simulink model "inloop_tf_model_spring"  (R2020b)
settings: Solver=VariableStepAuto  StartTime=0.0  StopTime=10.0  RelTol=1e-3
undefined symbols (not defined in the file or in its folder): b, ct, g, Jm, Ke, Kt, L, m, Rm
libraries: shared6dof x1
settings Model: Creator=Josh_  LastModifiedBy=Josh_

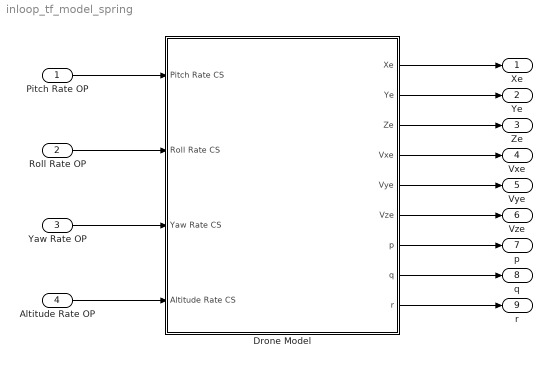
== system inloop_tf_model_spring ==
  Pitch Rate OP : Inport
  Roll Rate OP : Inport  Port=2
  Yaw Rate OP : Inport  Port=3
  Altitude Rate OP : Inport  Port=4
  Drone Model : Subsystem
  Xe : Outport
  Ye : Outport  Port=2
  Ze : Outport  Port=3
  Vxe : Outport  Port=4
  Vye : Outport  Port=5
  Vze : Outport  Port=6
  p : Outport  Port=7
  q : Outport  Port=8
  r : Outport  Port=9
  wires:
  Pitch Rate OP/1 -> Drone Model/1(Pitch Rate CS)
  Drone Model/9(r) -> r/1
  Roll Rate OP/1 -> Drone Model/2(Roll Rate CS)
  Drone Model/7(p) -> p/1
  Drone Model/4(Vxe) -> Vxe/1
  Drone Model/2(Ye) -> Ye/1
  Drone Model/3(Ze) -> Ze/1
  Altitude Rate OP/1 -> Drone Model/4(Altitude Rate CS)
  Drone Model/8(q) -> q/1
  Drone Model/6(Vze) -> Vze/1
  Drone Model/5(Vye) -> Vye/1
  Drone Model/1(Xe) -> Xe/1
  Yaw Rate OP/1 -> Drone Model/3(Yaw Rate CS)

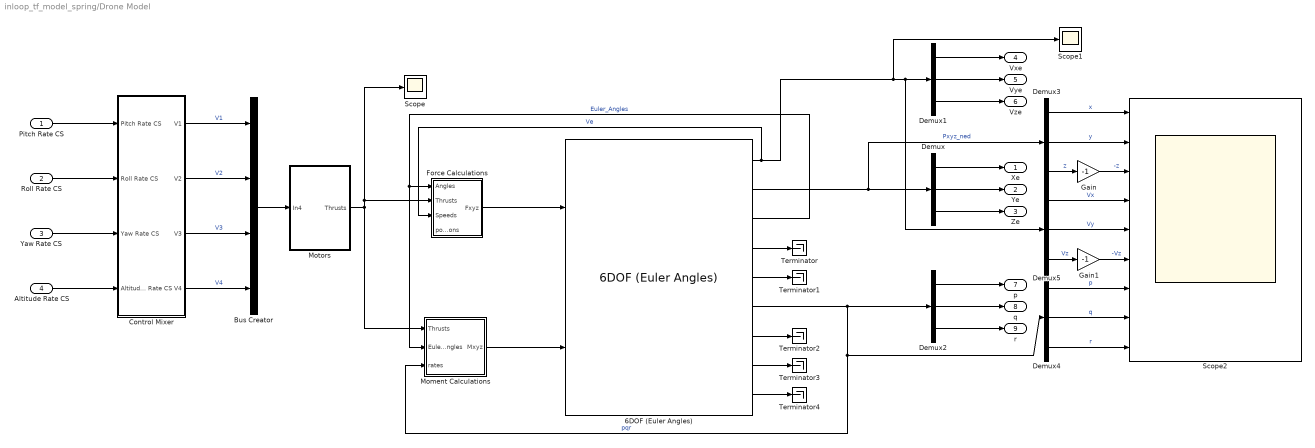
== system inloop_tf_model_spring/Drone Model ==
  Pitch Rate CS : Inport
  Roll Rate CS : Inport  Port=2
  Yaw Rate CS : Inport  Port=3
  Altitude Rate CS : Inport  Port=4
  6DOF (Euler Angles) : shared6dof/6DOF (Euler Angles)  units=Metric (MKS)  mtype=Fixed  rep=Euler Angles  xme_0=[0 0 0]  Vm_0=[0 0 0]  eul_0=[0 0 0]  pm_0=[0 0 0]  mass_0=m  mass_e=0.5  mass_f=2.0  inertia=eye(3)  inertia_e=eye(3)  inertia_f=2*eye(3)  k_quat=1.0  vre_flag=on  abi_flag=on  aMode=0  xme_statename=''  Vm_statename=''  eul_statename=''  quat_statename=''  pm_statename=''  mass_statename=''
      settings: SourceProductBaseCode=AE,PW,MT,UV,VE,VP
  Bus Creator : BusCreator  Inputs=4
  Control Mixer : Subsystem
  Demux{,1..5} (6 alike) : Demux  Outputs=3
  Force Calculations : Subsystem
  Gain : Gain  Gain=-1
  Gain1 : Gain  Gain=-1
  Moment Calculations : Subsystem
  Motors : Subsystem
  Scope : Scope
  Scope1 : Scope
  Scope2 : Scope  NumInputPorts=9
  Terminator{,1..4} (5 alike) : Terminator
  Xe : Outport
  Ye : Outport  Port=2
  Ze : Outport  Port=3
  Vxe : Outport  Port=4
  Vye : Outport  Port=5
  Vze : Outport  Port=6
  p : Outport  Port=7
  q : Outport  Port=8
  r : Outport  Port=9
  wires:
  6DOF (Euler Angles)/3 -> Moment Calculations/2(Euler Angles), Force Calculations/1(Angles)  "Euler_Angles"
  Demux1/3 -> Vze/1
  Demux5/1 -> Scope2/4  "Vx"
  6DOF (Euler Angles)/8 -> Terminator3/1
  6DOF (Euler Angles)/4 -> Terminator/1
  6DOF (Euler Angles)/7 -> Terminator2/1
  Demux4/3 -> Scope2/9  "r"
  Demux3/3 -> Gain/1  "z"
  Demux2/1 -> p/1
  6DOF (Euler Angles)/1 -> Force Calculations/3(Speeds), Demux5/1, Demux1/1, Scope1/1  "Ve"
  Demux5/3 -> Gain1/1  "Vz"
  Demux2/3 -> r/1
  Demux3/1 -> Scope2/1  "x"
  Force Calculations/1(Fxyz) -> 6DOF (Euler Angles)/1
  Demux1/2 -> Vye/1
  6DOF (Euler Angles)/6 -> Moment Calculations/3(rates), Demux4/1, Demux2/1  "pqr"
  Control Mixer/3(V3) -> Bus Creator/3  "V3"
  Demux4/1 -> Scope2/7  "p"
  Demux1/1 -> Vxe/1
  Demux/3 -> Ze/1
  Demux/2 -> Ye/1
  Demux/1 -> Xe/1
  Demux3/2 -> Scope2/2  "y"
  6DOF (Euler Angles)/5 -> Terminator1/1
  Demux4/2 -> Scope2/8  "q"
  Demux5/2 -> Scope2/5  "Vy"
  6DOF (Euler Angles)/9 -> Terminator4/1
  Demux2/2 -> q/1
  Motors/1(Thrusts) -> Scope/1, Force Calculations/2(Thrusts), Moment Calculations/1(Thrusts)
  6DOF (Euler Angles)/2 -> Demux/1, Demux3/1  "Pxyz_ned"
  Bus Creator/1 -> Motors/1(In4)
  Control Mixer/1(V1) -> Bus Creator/1  "V1"
  Moment Calculations/1(Mxyz) -> 6DOF (Euler Angles)/2
  Control Mixer/2(V2) -> Bus Creator/2  "V2"
  Control Mixer/4(V4) -> Bus Creator/4  "V4"
  Pitch Rate CS/1 -> Control Mixer/1(Pitch Rate CS)
  Roll Rate CS/1 -> Control Mixer/2(Roll Rate CS)
  Yaw Rate CS/1 -> Control Mixer/3(Yaw Rate CS)
  Altitude Rate CS/1 -> Control Mixer/4(Altitude Rate CS)
  Gain/1 -> Scope2/3  "-z"
  Gain1/1 -> Scope2/6  "-Vz"

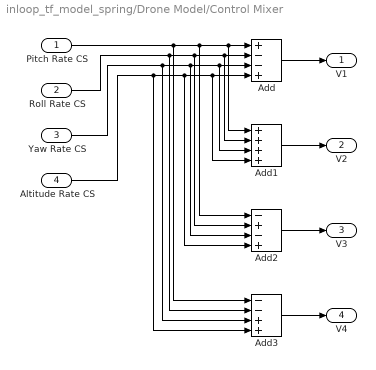
== system inloop_tf_model_spring/Drone Model/Control Mixer ==
  Pitch Rate CS : Inport
  Roll Rate CS : Inport  Port=2
  Yaw Rate CS : Inport  Port=3
  Altitude Rate CS : Inport  Port=4
  Add : Sum  Inputs=+--+
  Add1 : Sum  Inputs=++++
  Add2 : Sum  Inputs=-+-+
  Add3 : Sum  Inputs=--++
  V1 : Outport
  V2 : Outport  Port=2
  V3 : Outport  Port=3
  V4 : Outport  Port=4
  wires:
  Pitch Rate CS/1 -> Add1/1, Add/1, Add2/1, Add3/1
  Roll Rate CS/1 -> Add1/2, Add/2, Add2/2, Add3/2
  Yaw Rate CS/1 -> Add3/3, Add1/3, Add/3, Add2/3
  Altitude Rate CS/1 -> Add2/4, Add1/4, Add/4, Add3/4
  Add/1 -> V1/1
  Add1/1 -> V2/1
  Add2/1 -> V3/1
  Add3/1 -> V4/1

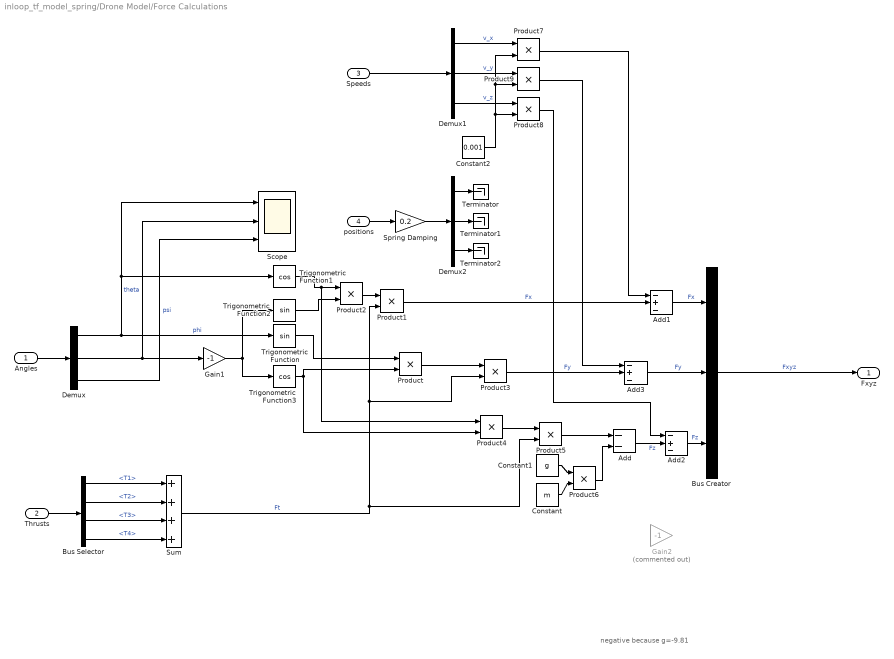
== system inloop_tf_model_spring/Drone Model/Force Calculations ==
  note: negative because g=-9.81
  Angles : Inport
  Thrusts : Inport  Port=2
  Speeds : Inport  Port=3
  positions : Inport  Port=4
  Add : Sum  Inputs=--
  Add1 : Sum  Inputs=-+-
  Add2 : Sum  Inputs=-+-
  Add3 : Sum  Inputs=-+-
  Bus Creator : BusCreator  Inputs=3
  Bus Selector : BusSelector  OutputSignals=T1,T2,T3,T4
  Constant : Constant  Value=m
  Constant1 : Constant  Value=g
  Constant2 : Constant  Value=0.001
  Demux : Demux  Outputs=3
  Demux1 : Demux  Outputs=3
  Demux2 : Demux  Outputs=3
  Gain1 : Gain  Gain=-1
  Gain2 : Gain  Commented=on  Gain=-1
  Product{,1..9} (10 alike) : Product
  Scope : Scope  NumInputPorts=3
  Spring Damping : Gain  Gain=0.2
  Sum : Sum  Inputs=++++
  Terminator : Terminator
  Terminator1 : Terminator
  Terminator2 : Terminator
  Trigonometric Function : Trigonometry
  Trigonometric Function1 : Trigonometry  Operator=cos
  Trigonometric Function2 : Trigonometry
  Trigonometric Function3 : Trigonometry  Operator=cos
  Fxyz : Outport
  wires:
  Constant/1 -> Product6/2
  Constant1/1 -> Product6/1
  Product5/1 -> Add/1
  Product4/1 -> Product5/1
  Product/1 -> Product3/1
  Demux/2 -> Gain1/1, Scope/2  "theta"
  Demux/1 -> Trigonometric Function/1, Trigonometric Function1/1, Scope/1  "phi"
  Angles/1 -> Demux/1
  Demux/3 -> Scope/3  "psi"
  Gain1/1 -> Trigonometric Function2/1, Trigonometric Function3/1
  Trigonometric Function1/1 -> Product4/1, Product2/1
  Trigonometric Function2/1 -> Product2/2
  Product2/1 -> Product1/1
  Sum/1 -> Product5/2, Product1/2, Product3/2  "Ft"
  Trigonometric Function/1 -> Product/1
  Trigonometric Function3/1 -> Product4/2, Product/2
  Thrusts/1 -> Bus Selector/1
  Bus Selector/1 -> Sum/1  "<T1>"
  Bus Selector/2 -> Sum/2  "<T2>"
  Bus Selector/3 -> Sum/3  "<T3>"
  Bus Selector/4 -> Sum/4  "<T4>"
  Bus Creator/1 -> Fxyz/1  "Fxyz"
  Product6/1 -> Add/2
  Speeds/1 -> Demux1/1
  Demux1/1 -> Product7/1  "v_x"
  Demux1/2 -> Product9/1  "v_y"
  Demux1/3 -> Product8/1  "v_z"
  Constant2/1 -> Product8/2, Product9/2, Product7/2
  Product1/1 -> Add1/2  "Fx"
  Add1/1 -> Bus Creator/1  "Fx"
  Add/1 -> Add2/2  "Fz"
  Add2/1 -> Bus Creator/3  "Fz"
  Add3/1 -> Bus Creator/2  "Fy"
  Product3/1 -> Add3/2  "Fy"
  Product8/1 -> Add2/1
  Product9/1 -> Add3/1
  Product7/1 -> Add1/1
  positions/1 -> Spring Damping/1
  Spring Damping/1 -> Demux2/1
  Demux2/1 -> Terminator/1
  Demux2/3 -> Terminator2/1
  Demux2/2 -> Terminator1/1

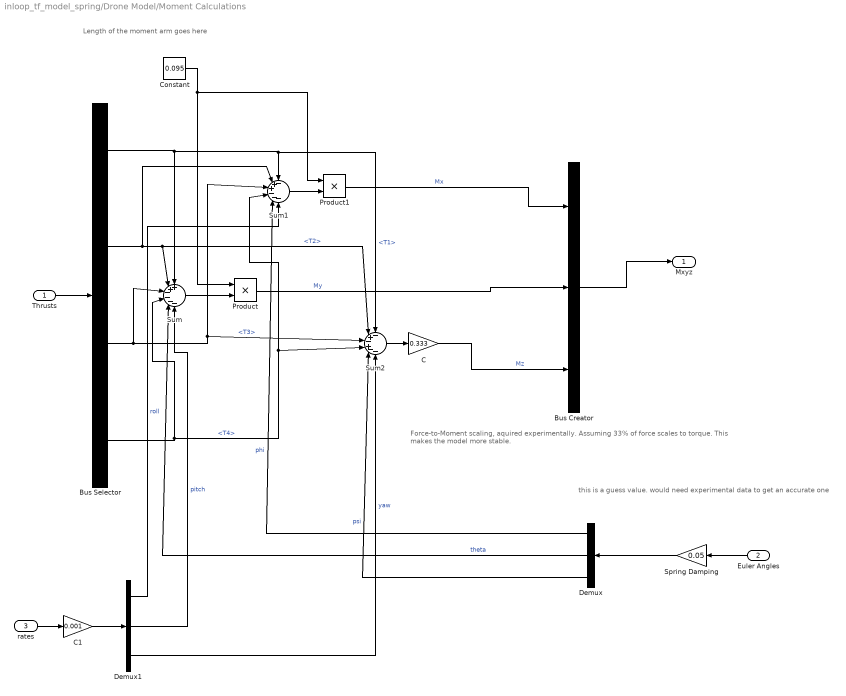
== system inloop_tf_model_spring/Drone Model/Moment Calculations ==
  note: this is a guess value. would need experimental data to get an accurate one
  note: Length of the moment arm goes here
  note: Force-to-Moment scaling, aquired experimentally. Assuming 33% of force scales to torque. This makes the model more stable.
  Thrusts : Inport
  Euler Angles : Inport  Port=2
  rates : Inport  Port=3
  Bus Creator : BusCreator  Inputs=3
  Bus Selector : BusSelector  OutputSignals=T1,T2,T3,T4
  C : Gain  Gain=0.333
  C1 : Gain  Gain=0.001
  Constant : Constant  Value=0.095
  Demux : Demux  Outputs=3
  Demux1 : Demux  Outputs=3
  Product : Product
  Product1 : Product
  Spring Damping : Gain  Gain=0.05
  Sum : Sum  Inputs=++----
  Sum1 : Sum  Inputs=-++---
  Sum2 : Sum  Inputs=-+-+--
  Mxyz : Outport
  wires:
  Bus Creator/1 -> Mxyz/1
  Bus Selector/1 -> Sum2/1, Sum1/1, Sum/1  "<T1>"
  Bus Selector/4 -> Sum2/4, Sum1/4, Sum/4  "<T4>"
  Thrusts/1 -> Bus Selector/1
  Bus Selector/2 -> Sum/2, Sum2/2, Sum1/2  "<T2>"
  Bus Selector/3 -> Sum1/3, Sum2/3, Sum/3  "<T3>"
  Sum2/1 -> C/1
  C/1 -> Bus Creator/3  "Mz"
  Sum/1 -> Product/2
  Constant/1 -> Product1/1, Product/1
  Sum1/1 -> Product1/2
  Product1/1 -> Bus Creator/1  "Mx"
  Product/1 -> Bus Creator/2  "My"
  Demux/1 -> Sum1/5  "phi"
  Demux/2 -> Sum/5  "theta"
  Demux/3 -> Sum2/5  "psi"
  Euler Angles/1 -> Spring Damping/1
  Spring Damping/1 -> Demux/1
  Demux1/2 -> Sum/6  "pitch"
  Demux1/3 -> Sum2/6  "yaw"
  Demux1/1 -> Sum1/6  "roll"
  rates/1 -> C1/1
  C1/1 -> Demux1/1

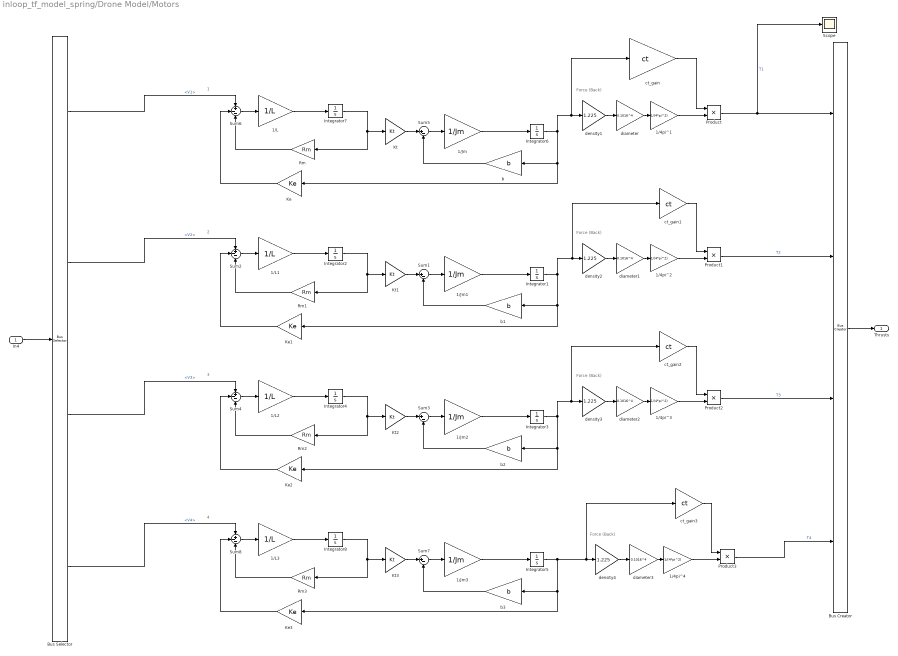
== system inloop_tf_model_spring/Drone Model/Motors ==
  note: Force (Back)
  note: 1
  note: 2
  note: Force (Back)
  note: 3
  note: Force (Back)
  note: 4
  note: Force (Back)
  In4 : Inport
  1/4pi^{1..4} (4 alike) : Gain  Gain=1/(4*pi^2)
  1/Jm{,1..3} (4 alike) : Gain  Gain=1/Jm
  1/L{,1..3} (4 alike) : Gain  Gain=1/L
  Bus Creator : BusCreator  Inputs=4
  Bus Selector : BusSelector  OutputSignals=V1,V2,V3,V4
  Integrator{1..8} (8 alike) : Integrator
  Ke{,1..3} (4 alike) : Gain  Gain=Ke
  Kt{,1..3} (4 alike) : Gain  Gain=Kt
  Product{,1..3} (4 alike) : Product
  Rm{,1..3} (4 alike) : Gain  Gain=Rm
  Scope : Scope
  Sum{1,3,5,7} (4 alike) : Sum  Inputs=|+-
  Sum{2,4,6,8} (4 alike) : Sum  Inputs=+--
  b{,1..3} (4 alike) : Gain  Gain=b
  ct_gain{,1..3} (4 alike) : Gain  Gain=ct
  density{1..4} (4 alike) : Gain  Gain=1.225
  diameter{,1..3} (4 alike) : Gain  Gain=0.1016^4
  Thrusts : Outport
  wires:
  In4/1 -> Bus Selector/1
  Sum5/1 -> 1/Jm/1
  Rm/1 -> Sum6/3
  1/Jm/1 -> Integrator6/1
  1/L/1 -> Integrator7/1
  diameter/1 -> 1/4pi^1/1
  Integrator6/1 -> density1/1, ct_gain/1, b/1, Ke/1
  1/4pi^1/1 -> Product/2
  Integrator7/1 -> Rm/1, Kt/1
  Kt/1 -> Sum5/1
  density1/1 -> diameter/1
  b/1 -> Sum5/2
  Sum6/1 -> 1/L/1
  Ke/1 -> Sum6/2
  Bus Creator/1 -> Thrusts/1
  b1/1 -> Sum1/2
  Ke1/1 -> Sum2/2
  Integrator2/1 -> Rm1/1, Kt1/1
  density2/1 -> diameter1/1
  Sum2/1 -> 1/L1/1
  1/4pi^2/1 -> Product1/2
  1/Jm1/1 -> Integrator1/1
  diameter1/1 -> 1/4pi^2/1
  Kt1/1 -> Sum1/1
  1/L1/1 -> Integrator2/1
  Rm1/1 -> Sum2/3
  Sum1/1 -> 1/Jm1/1
  b2/1 -> Sum3/2
  Ke2/1 -> Sum4/2
  Integrator4/1 -> Rm2/1, Kt2/1
  density3/1 -> diameter2/1
  Sum4/1 -> 1/L2/1
  1/4pi^3/1 -> Product2/2
  1/Jm2/1 -> Integrator3/1
  diameter2/1 -> 1/4pi^3/1
  Kt2/1 -> Sum3/1
  1/L2/1 -> Integrator4/1
  Rm2/1 -> Sum4/3
  Sum3/1 -> 1/Jm2/1
  b3/1 -> Sum7/2
  Ke3/1 -> Sum8/2
  Integrator8/1 -> Rm3/1, Kt3/1
  density4/1 -> diameter3/1
  Sum8/1 -> 1/L3/1
  1/4pi^4/1 -> Product3/2
  1/Jm3/1 -> Integrator5/1
  diameter3/1 -> 1/4pi^4/1
  Kt3/1 -> Sum7/1
  1/L3/1 -> Integrator8/1
  Rm3/1 -> Sum8/3
  Sum7/1 -> 1/Jm3/1
  ct_gain/1 -> Product/1
  Product/1 -> Scope/1, Bus Creator/1  "T1"
  Product1/1 -> Bus Creator/2  "T2"
  Product2/1 -> Bus Creator/3  "T3"
  Product3/1 -> Bus Creator/4  "T4"
  Integrator1/1 -> ct_gain1/1, density2/1, b1/1, Ke1/1
  ct_gain1/1 -> Product1/1
  Integrator3/1 -> ct_gain2/1, density3/1, b2/1, Ke2/1
  ct_gain2/1 -> Product2/1
  Integrator5/1 -> b3/1, Ke3/1, ct_gain3/1, density4/1
  ct_gain3/1 -> Product3/1
  Bus Selector/1 -> Sum6/1  "<V1>"
  Bus Selector/2 -> Sum2/1  "<V2>"
  Bus Selector/3 -> Sum4/1  "<V3>"
  Bus Selector/4 -> Sum8/1  "<V4>"
